simulink model "iot_casestudy_1_32"  (R2023a)
settings: Solver=VariableStepAuto  StartTime=0.0  StopTime=3.0  RelTol=1e-3
undefined symbols (not defined in the file or in its folder): m, n
(part 2 of 3)

== stateflow chart iot_casestudy_1_32/CameraScheduler4 ==
  settings: updateMethod=CONTINUOUS  executeAtInitialization=1
  state Main
    entry:
    dt=timer_array[i];
  (default) -> Main : {i=1;dt=0;}
  Main -> Main : after(dt,msec){i=i+1;send(schedule_driver);send(schedule_control);}
  data: timer_array input; schedule_driver output double; schedule_control output double; dt local double; dt2 local double; i output double =0.0

== stateflow chart iot_casestudy_1_32/CameraScheduler5 ==
  settings: updateMethod=CONTINUOUS  executeAtInitialization=1
  state Main
    entry:
    dt=timer_array[i];
  (default) -> Main : {i=0;dt=0;}
  Main -> Main : after(dt,msec){i=i+1;send(schedule_driver);send(schedule_control);}
  data: timer_array input; i local double; schedule_driver output double; schedule_control output double; dt local double

== stateflow chart iot_casestudy_1_32/CameraScheduler6 ==
  settings: updateMethod=CONTINUOUS  executeAtInitialization=1
  state Main
    entry:
    dt=timer_array[i];
  (default) -> Main : {i=1;dt=0;}
  Main -> Main : after(dt,msec){i=i+1;send(schedule_driver);send(schedule_control);}
  data: timer_array input; schedule_driver output double; schedule_control output double; dt local double; dt2 local double; i output double =0.0

== stateflow chart iot_casestudy_1_32/CameraScheduler7 ==
  settings: updateMethod=CONTINUOUS  executeAtInitialization=1
  state Main
    entry:
    dt=timer_array[i];
  (default) -> Main : {i=0;dt=0;}
  Main -> Main : after(dt,msec){i=i+1;send(schedule_driver);send(schedule_control);}
  data: timer_array input; i local double; schedule_driver output double; schedule_control output double; dt local double

== stateflow chart iot_casestudy_1_32/CameraControl10 ==
  settings: updateMethod=CONTINUOUS
  state Operation
    state RequestHangling [parallel]
      settings: executionOrder=1
      state Operation1
      (default) -> Operation1 : {image_request=1;}
      Operation1 -> Operation1 : schedule{image_request=1;}
    state ImageMessaging [parallel]
      settings: executionOrder=2
      state Operation2
        entry:
        validity=isvalid(imageIn);
      (default) -> Operation2 : {i=1;}
      (junction 28) -> Operation2 [order 1] : [validity==1]
          | {receive(imageIn);i = i + 1;
          | imageOut.data=imageIn.data
          | send(imageOut);}
      (junction 28) -> Operation2 [order 2] : {i = i + 1;receive(imageIn);}
      (junction 19) -> (junction 28) [order 1] : [network_faults(i)==0]
      (junction 19) -> Operation2 [order 2] : {receive(imageIn);i = i + 1;}
      Operation2 -> (junction 19) : schedule
  (default) -> Operation
  data: image_request output; imageIn input; i local; network_faults input; imageOut output; schedule input; validity local

== stateflow chart iot_casestudy_1_32/CameraControl11 ==
  settings: updateMethod=CONTINUOUS
  state Operation
    state RequestHangling [parallel]
      settings: executionOrder=1
      note: {image_request=1;}
      state Operation1
      (default) -> Operation1
      Operation1 -> Operation1 : schedule{image_request=1;}
    state ImageMessaging [parallel]
      settings: executionOrder=2
      state Operation2
        entry:
        validity=isvalid(imageIn);
      (default) -> Operation2 : {i=1;}
      (junction 29) -> Operation2 [order 1] : [isvalid(imageIn)==1]
          | {receive(imageIn);i = i + 1;
          | imageOut.data=imageIn.data;
          | send(imageOut);}
      (junction 19) -> Operation2 [order 2] : {receive(imageIn);i = i + 1;}
      Operation2 -> (junction 19) : schedule
      (junction 29) -> Operation2 [order 2] : {i = i + 1;receive(imageIn);}
      (junction 19) -> (junction 29) [order 1] : [network_faults(i)==0]
  (default) -> Operation
  data: image_request output; imageIn input; i local; network_faults input; imageOut output; schedule input; validity local

== stateflow chart iot_casestudy_1_32/CameraControl12 ==
  settings: updateMethod=CONTINUOUS
  state Operation
    state RequestHangling [parallel]
      settings: executionOrder=1
      state Operation1
      (default) -> Operation1 : {image_request=1;}
      Operation1 -> Operation1 : schedule{image_request=1;}
    state ImageMessaging [parallel]
      settings: executionOrder=2
      state Operation2
        entry:
        validity=isvalid(imageIn);
      (default) -> Operation2 : {i=1;}
      (junction 28) -> Operation2 [order 1] : [validity==1]
          | {receive(imageIn);i = i + 1;
          | imageOut.data=imageIn.data
          | send(imageOut);}
      (junction 28) -> Operation2 [order 2] : {i = i + 1;receive(imageIn);}
      (junction 19) -> (junction 28) [order 1] : [network_faults(i)==0]
      (junction 19) -> Operation2 [order 2] : {receive(imageIn);i = i + 1;}
      Operation2 -> (junction 19) : schedule
  (default) -> Operation
  data: image_request output; imageIn input; i local; network_faults input; imageOut output; schedule input; validity local

== stateflow chart iot_casestudy_1_32/CameraControl13 ==
  settings: updateMethod=CONTINUOUS
  state Operation
    state RequestHangling [parallel]
      settings: executionOrder=1
      note: {image_request=1;}
      state Operation1
      (default) -> Operation1
      Operation1 -> Operation1 : schedule{image_request=1;}
    state ImageMessaging [parallel]
      settings: executionOrder=2
      state Operation2
        entry:
        validity=isvalid(imageIn);
      (default) -> Operation2 : {i=1;}
      (junction 29) -> Operation2 [order 1] : [isvalid(imageIn)==1]
          | {receive(imageIn);i = i + 1;
          | imageOut.data=imageIn.data;
          | send(imageOut);}
      (junction 19) -> Operation2 [order 2] : {receive(imageIn);i = i + 1;}
      Operation2 -> (junction 19) : schedule
      (junction 29) -> Operation2 [order 2] : {i = i + 1;receive(imageIn);}
      (junction 19) -> (junction 29) [order 1] : [network_faults(i)==0]
  (default) -> Operation
  data: image_request output; imageIn input; i local; network_faults input; imageOut output; schedule input; validity local

== stateflow chart iot_casestudy_1_32/CameraControl14 ==
  settings: updateMethod=CONTINUOUS
  state Operation
    state RequestHangling [parallel]
      settings: executionOrder=1
      state Operation1
      (default) -> Operation1 : {image_request=1;}
      Operation1 -> Operation1 : schedule{image_request=1;}
    state ImageMessaging [parallel]
      settings: executionOrder=2
      state Operation2
        entry:
        validity=isvalid(imageIn);
      (default) -> Operation2 : {i=1;}
      (junction 28) -> Operation2 [order 1] : [validity==1]
          | {receive(imageIn);i = i + 1;
          | imageOut.data=imageIn.data
          | send(imageOut);}
      (junction 28) -> Operation2 [order 2] : {i = i + 1;receive(imageIn);}
      (junction 19) -> (junction 28) [order 1] : [network_faults(i)==0]
      (junction 19) -> Operation2 [order 2] : {receive(imageIn);i = i + 1;}
      Operation2 -> (junction 19) : schedule
  (default) -> Operation
  data: image_request output; imageIn input; i local; network_faults input; imageOut output; schedule input; validity local

== stateflow chart iot_casestudy_1_32/CameraControl15 ==
  settings: updateMethod=CONTINUOUS
  state Operation
    state RequestHangling [parallel]
      settings: executionOrder=1
      note: {image_request=1;}
      state Operation1
      (default) -> Operation1
      Operation1 -> Operation1 : schedule{image_request=1;}
    state ImageMessaging [parallel]
      settings: executionOrder=2
      state Operation2
        entry:
        validity=isvalid(imageIn);
      (default) -> Operation2 : {i=1;}
      (junction 29) -> Operation2 [order 1] : [isvalid(imageIn)==1]
          | {receive(imageIn);i = i + 1;
          | imageOut.data=imageIn.data;
          | send(imageOut);}
      (junction 19) -> Operation2 [order 2] : {receive(imageIn);i = i + 1;}
      Operation2 -> (junction 19) : schedule
      (junction 29) -> Operation2 [order 2] : {i = i + 1;receive(imageIn);}
      (junction 19) -> (junction 29) [order 1] : [network_faults(i)==0]
  (default) -> Operation
  data: image_request output; imageIn input; i local; network_faults input; imageOut output; schedule input; validity local

== stateflow chart iot_casestudy_1_32/CameraControl8 ==
  settings: updateMethod=CONTINUOUS
  state Operation
    state RequestHangling [parallel]
      settings: executionOrder=1
      state Operation1
      (default) -> Operation1 : {image_request=1;}
      Operation1 -> Operation1 : schedule{image_request=1;}
    state ImageMessaging [parallel]
      settings: executionOrder=2
      state Operation2
        entry:
        validity=isvalid(imageIn);
      (default) -> Operation2 : {i=1;}
      (junction 28) -> Operation2 [order 1] : [validity==1]
          | {receive(imageIn);i = i + 1;
          | imageOut.data=imageIn.data
          | send(imageOut);}
      (junction 28) -> Operation2 [order 2] : {i = i + 1;receive(imageIn);}
      (junction 19) -> (junction 28) [order 1] : [network_faults(i)==0]
      (junction 19) -> Operation2 [order 2] : {receive(imageIn);i = i + 1;}
      Operation2 -> (junction 19) : schedule
  (default) -> Operation
  data: image_request output; imageIn input; i local; network_faults input; imageOut output; schedule input; validity local

== stateflow chart iot_casestudy_1_32/CameraControl9 ==
  settings: updateMethod=CONTINUOUS
  state Operation
    state RequestHangling [parallel]
      settings: executionOrder=1
      note: {image_request=1;}
      state Operation1
      (default) -> Operation1
      Operation1 -> Operation1 : schedule{image_request=1;}
    state ImageMessaging [parallel]
      settings: executionOrder=2
      state Operation2
        entry:
        validity=isvalid(imageIn);
      (default) -> Operation2 : {i=1;}
      (junction 29) -> Operation2 [order 1] : [isvalid(imageIn)==1]
          | {receive(imageIn);i = i + 1;
          | imageOut.data=imageIn.data;
          | send(imageOut);}
      (junction 19) -> Operation2 [order 2] : {receive(imageIn);i = i + 1;}
      Operation2 -> (junction 19) : schedule
      (junction 29) -> Operation2 [order 2] : {i = i + 1;receive(imageIn);}
      (junction 19) -> (junction 29) [order 1] : [network_faults(i)==0]
  (default) -> Operation
  data: image_request output; imageIn input; i local; network_faults input; imageOut output; schedule input; validity local

== stateflow chart iot_casestudy_1_32/CameraDriver10 ==
  settings: updateMethod=CONTINUOUS
  state Operation
    state CarVisibility [parallel]
      settings: executionOrder=1
      state NoCar
        entry: car=0;
      state Car
        entry: car=1;
      (default) -> NoCar
      NoCar -> Car : [traffic_state==1]
      Car -> NoCar : [traffic_state==0]
    state DriverOperation [parallel]
      settings: executionOrder=2
      state Main
      (default) -> Main : {i=1;}
      Main -> (junction 22) : schedule[image_request]
      (junction 22) -> Main [order 2] : {image.data=0;
          | send(image);i = i + 1;}
      (junction 22) -> Main [order 1] : [(car==1)&&(blurryness(i)==1)]
          | {image.data=1;i = i + 1;send(image);}
  data: image_request input; traffic_state input; blurryness input; image output; car local; i local; schedule input

== stateflow chart iot_casestudy_1_32/CameraDriver11 ==
  settings: updateMethod=CONTINUOUS
  state Operation
    state CarVisibility [parallel]
      settings: executionOrder=1
      state NoCar
        entry: car=0;
      state Car
        entry: car=1;
      (default) -> NoCar
      NoCar -> Car : [traffic_state==1]
      Car -> NoCar : [traffic_state==0]
    state DriverOperation [parallel]
      settings: executionOrder=2
      state Main
      (default) -> Main : {i=1;}
      Main -> (junction 22) : schedule
          | [image_request]
      (junction 22) -> Main [order 1] : [(car==1)&&(blurryness(i)==1)]
          | {image.data=1;send(image);i = i + 1;}
      (junction 22) -> Main [order 2] : {image.data=0;
          | send(image);i = i + 1;}
  data: image_request input; traffic_state input; blurryness input; image output; car local; i local; schedule input

== stateflow chart iot_casestudy_1_32/CameraDriver12 ==
  settings: updateMethod=CONTINUOUS
  state Operation
    state CarVisibility [parallel]
      settings: executionOrder=1
      state NoCar
        entry: car=0;
      state Car
        entry: car=1;
      (default) -> NoCar
      NoCar -> Car : [traffic_state==1]
      Car -> NoCar : [traffic_state==0]
    state DriverOperation [parallel]
      settings: executionOrder=2
      state Main
      (default) -> Main : {i=1;}
      Main -> (junction 22) : schedule[image_request]
      (junction 22) -> Main [order 2] : {image.data=0;
          | send(image);i = i + 1;}
      (junction 22) -> Main [order 1] : [(car==1)&&(blurryness(i)==1)]
          | {image.data=1;i = i + 1;send(image);}
  data: image_request input; traffic_state input; blurryness input; image output; car local; i local; schedule input

== stateflow chart iot_casestudy_1_32/CameraDriver13 ==
  settings: updateMethod=CONTINUOUS
  state Operation
    state CarVisibility [parallel]
      settings: executionOrder=1
      state NoCar
        entry: car=0;
      state Car
        entry: car=1;
      (default) -> NoCar
      NoCar -> Car : [traffic_state==1]
      Car -> NoCar : [traffic_state==0]
    state DriverOperation [parallel]
      settings: executionOrder=2
      state Main
      (default) -> Main : {i=1;}
      Main -> (junction 22) : schedule
          | [image_request]
      (junction 22) -> Main [order 1] : [(car==1)&&(blurryness(i)==1)]
          | {image.data=1;send(image);i = i + 1;}
      (junction 22) -> Main [order 2] : {image.data=0;
          | send(image);i = i + 1;}
  data: image_request input; traffic_state input; blurryness input; image output; car local; i local; schedule input

== stateflow chart iot_casestudy_1_32/CameraDriver14 ==
  settings: updateMethod=CONTINUOUS
  state Operation
    state CarVisibility [parallel]
      settings: executionOrder=1
      state NoCar
        entry: car=0;
      state Car
        entry: car=1;
      (default) -> NoCar
      NoCar -> Car : [traffic_state==1]
      Car -> NoCar : [traffic_state==0]
    state DriverOperation [parallel]
      settings: executionOrder=2
      state Main
      (default) -> Main : {i=1;}
      Main -> (junction 22) : schedule[image_request]
      (junction 22) -> Main [order 2] : {image.data=0;
          | send(image);i = i + 1;}
      (junction 22) -> Main [order 1] : [(car==1)&&(blurryness(i)==1)]
          | {image.data=1;i = i + 1;send(image);}
  data: image_request input; traffic_state input; blurryness input; image output; car local; i local; schedule input

== stateflow chart iot_casestudy_1_32/CameraDriver15 ==
  settings: updateMethod=CONTINUOUS
  state Operation
    state CarVisibility [parallel]
      settings: executionOrder=1
      state NoCar
        entry: car=0;
      state Car
        entry: car=1;
      (default) -> NoCar
      NoCar -> Car : [traffic_state==1]
      Car -> NoCar : [traffic_state==0]
    state DriverOperation [parallel]
      settings: executionOrder=2
      state Main
      (default) -> Main : {i=1;}
      Main -> (junction 22) : schedule
          | [image_request]
      (junction 22) -> Main [order 1] : [(car==1)&&(blurryness(i)==1)]
          | {image.data=1;send(image);i = i + 1;}
      (junction 22) -> Main [order 2] : {image.data=0;
          | send(image);i = i + 1;}
  data: image_request input; traffic_state input; blurryness input; image output; car local; i local; schedule input

== stateflow chart iot_casestudy_1_32/CameraDriver8 ==
  settings: updateMethod=CONTINUOUS
  state Operation
    state CarVisibility [parallel]
      settings: executionOrder=1
      state NoCar
        entry: car=0;
      state Car
        entry: car=1;
      (default) -> NoCar
      NoCar -> Car : [traffic_state==1]
      Car -> NoCar : [traffic_state==0]
    state DriverOperation [parallel]
      settings: executionOrder=2
      state Main
      (default) -> Main : {i=1;}
      Main -> (junction 22) : schedule[image_request]
      (junction 22) -> Main [order 2] : {image.data=0;
          | send(image);i = i + 1;}
      (junction 22) -> Main [order 1] : [(car==1)&&(blurryness(i)==1)]
          | {image.data=1;i = i + 1;send(image);}
  data: image_request input; traffic_state input; blurryness input; image output; car local; i local; schedule input

== stateflow chart iot_casestudy_1_32/CameraDriver9 ==
  settings: updateMethod=CONTINUOUS
  state Operation
    state CarVisibility [parallel]
      settings: executionOrder=1
      state NoCar
        entry: car=0;
      state Car
        entry: car=1;
      (default) -> NoCar
      NoCar -> Car : [traffic_state==1]
      Car -> NoCar : [traffic_state==0]
    state DriverOperation [parallel]
      settings: executionOrder=2
      state Main
      (default) -> Main : {i=1;}
      Main -> (junction 22) : schedule
          | [image_request]
      (junction 22) -> Main [order 1] : [(car==1)&&(blurryness(i)==1)]
          | {image.data=1;send(image);i = i + 1;}
      (junction 22) -> Main [order 2] : {image.data=0;
          | send(image);i = i + 1;}
  data: image_request input; traffic_state input; blurryness input; image output; car local; i local; schedule input

== stateflow chart iot_casestudy_1_32/CameraScheduler10 ==
  settings: updateMethod=CONTINUOUS  executeAtInitialization=1
  state Main
    entry:
    dt=timer_array[i];
  (default) -> Main : {i=1;dt=0;}
  Main -> Main : after(dt,msec){i=i+1;send(schedule_driver);send(schedule_control);}
  data: timer_array input; schedule_driver output double; schedule_control output double; dt local double; dt2 local double; i local double =0.0

== stateflow chart iot_casestudy_1_32/CameraScheduler11 ==
  settings: updateMethod=CONTINUOUS  executeAtInitialization=1
  state Main
    entry:
    dt=timer_array[i];
  (default) -> Main : {i=0;dt=0;}
  Main -> Main : after(dt,msec){i=i+1;send(schedule_driver);send(schedule_control);}
  data: timer_array input; i local double; schedule_driver output double; schedule_control output double; dt local double

== stateflow chart iot_casestudy_1_32/CameraScheduler12 ==
  settings: updateMethod=CONTINUOUS  executeAtInitialization=1
  state Main
    entry:
    dt=timer_array[i];
  (default) -> Main : {i=1;dt=0;}
  Main -> Main : after(dt,msec){i=i+1;send(schedule_driver);send(schedule_control);}
  data: timer_array input; schedule_driver output double; schedule_control output double; dt local double; dt2 local double; i local double =0.0

== stateflow chart iot_casestudy_1_32/CameraScheduler13 ==
  settings: updateMethod=CONTINUOUS  executeAtInitialization=1
  state Main
    entry:
    dt=timer_array[i];
  (default) -> Main : {i=0;dt=0;}
  Main -> Main : after(dt,msec){i=i+1;send(schedule_driver);send(schedule_control);}
  data: timer_array input; i local double; schedule_driver output double; schedule_control output double; dt local double

== stateflow chart iot_casestudy_1_32/CameraScheduler14 ==
  settings: updateMethod=CONTINUOUS  executeAtInitialization=1
  state Main
    entry:
    dt=timer_array[i];
  (default) -> Main : {i=1;dt=0;}
  Main -> Main : after(dt,msec){i=i+1;send(schedule_driver);send(schedule_control);}
  data: timer_array input; schedule_driver output double; schedule_control output double; dt local double; dt2 local double; i local double =0.0

== stateflow chart iot_casestudy_1_32/CameraScheduler15 ==
  settings: updateMethod=CONTINUOUS  executeAtInitialization=1
  state Main
    entry:
    dt=timer_array[i];
  (default) -> Main : {i=0;dt=0;}
  Main -> Main : after(dt,msec){i=i+1;send(schedule_driver);send(schedule_control);}
  data: timer_array input; i local double; schedule_driver output double; schedule_control output double; dt local double

== stateflow chart iot_casestudy_1_32/CameraScheduler8 ==
  settings: updateMethod=CONTINUOUS  executeAtInitialization=1
  state Main
    entry:
    dt=timer_array[i];
  (default) -> Main : {i=1;dt=0;}
  Main -> Main : after(dt,msec){i=i+1;send(schedule_driver);send(schedule_control);}
  data: timer_array input; schedule_driver output double; schedule_control output double; dt local double; dt2 local double; i local double =0.0

== stateflow chart iot_casestudy_1_32/CameraScheduler9 ==
  settings: updateMethod=CONTINUOUS  executeAtInitialization=1
  state Main
    entry:
    dt=timer_array[i];
  (default) -> Main : {i=0;dt=0;}
  Main -> Main : after(dt,msec){i=i+1;send(schedule_driver);send(schedule_control);}
  data: timer_array input; i local double; schedule_driver output double; schedule_control output double; dt local double

== stateflow chart iot_casestudy_1_32/CameraControl16 ==
  settings: updateMethod=CONTINUOUS
  state Operation
    state RequestHangling [parallel]
      settings: executionOrder=1
      state Operation1
      (default) -> Operation1 : {image_request=1;}
      Operation1 -> Operation1 : schedule{image_request=1;}
    state ImageMessaging [parallel]
      settings: executionOrder=2
      state Operation2
        entry:
        validity=isvalid(imageIn);
      (default) -> Operation2 : {i=1;}
      (junction 28) -> Operation2 [order 1] : [validity==1]
          | {receive(imageIn);i = i + 1;
          | imageOut.data=imageIn.data
          | send(imageOut);}
      (junction 28) -> Operation2 [order 2] : {i = i + 1;receive(imageIn);}
      (junction 19) -> (junction 28) [order 1] : [network_faults(i)==0]
      (junction 19) -> Operation2 [order 2] : {receive(imageIn);i = i + 1;}
      Operation2 -> (junction 19) : schedule
  (default) -> Operation
  data: image_request output; imageIn input; i local; network_faults input; imageOut output; schedule input; validity local

== stateflow chart iot_casestudy_1_32/CameraControl17 ==
  settings: updateMethod=CONTINUOUS
  state Operation
    state RequestHangling [parallel]
      settings: executionOrder=1
      note: {image_request=1;}
      state Operation1
      (default) -> Operation1
      Operation1 -> Operation1 : schedule{image_request=1;}
    state ImageMessaging [parallel]
      settings: executionOrder=2
      state Operation2
        entry:
        validity=isvalid(imageIn);
      (default) -> Operation2 : {i=1;}
      (junction 29) -> Operation2 [order 1] : [isvalid(imageIn)==1]
          | {receive(imageIn);i = i + 1;
          | imageOut.data=imageIn.data;
          | send(imageOut);}
      (junction 19) -> Operation2 [order 2] : {receive(imageIn);i = i + 1;}
      Operation2 -> (junction 19) : schedule
      (junction 29) -> Operation2 [order 2] : {i = i + 1;receive(imageIn);}
      (junction 19) -> (junction 29) [order 1] : [network_faults(i)==0]
  (default) -> Operation
  data: image_request output; imageIn input; i local; network_faults input; imageOut output; schedule input; validity local

== stateflow chart iot_casestudy_1_32/CameraControl18 ==
  settings: updateMethod=CONTINUOUS
  state Operation
    state RequestHangling [parallel]
      settings: executionOrder=1
      state Operation1
      (default) -> Operation1 : {image_request=1;}
      Operation1 -> Operation1 : schedule{image_request=1;}
    state ImageMessaging [parallel]
      settings: executionOrder=2
      state Operation2
        entry:
        validity=isvalid(imageIn);
      (default) -> Operation2 : {i=1;}
      (junction 28) -> Operation2 [order 1] : [validity==1]
          | {receive(imageIn);i = i + 1;
          | imageOut.data=imageIn.data
          | send(imageOut);}
      (junction 28) -> Operation2 [order 2] : {i = i + 1;receive(imageIn);}
      (junction 19) -> (junction 28) [order 1] : [network_faults(i)==0]
      (junction 19) -> Operation2 [order 2] : {receive(imageIn);i = i + 1;}
      Operation2 -> (junction 19) : schedule
  (default) -> Operation
  data: image_request output; imageIn input; i local; network_faults input; imageOut output; schedule input; validity local

== stateflow chart iot_casestudy_1_32/CameraControl19 ==
  settings: updateMethod=CONTINUOUS
  state Operation
    state RequestHangling [parallel]
      settings: executionOrder=1
      note: {image_request=1;}
      state Operation1
      (default) -> Operation1
      Operation1 -> Operation1 : schedule{image_request=1;}
    state ImageMessaging [parallel]
      settings: executionOrder=2
      state Operation2
        entry:
        validity=isvalid(imageIn);
      (default) -> Operation2 : {i=1;}
      (junction 29) -> Operation2 [order 1] : [isvalid(imageIn)==1]
          | {receive(imageIn);i = i + 1;
          | imageOut.data=imageIn.data;
          | send(imageOut);}
      (junction 19) -> Operation2 [order 2] : {receive(imageIn);i = i + 1;}
      Operation2 -> (junction 19) : schedule
      (junction 29) -> Operation2 [order 2] : {i = i + 1;receive(imageIn);}
      (junction 19) -> (junction 29) [order 1] : [network_faults(i)==0]
  (default) -> Operation
  data: image_request output; imageIn input; i local; network_faults input; imageOut output; schedule input; validity local

== stateflow chart iot_casestudy_1_32/CameraControl20 ==
  settings: updateMethod=CONTINUOUS
  state Operation
    state RequestHangling [parallel]
      settings: executionOrder=1
      state Operation1
      (default) -> Operation1 : {image_request=1;}
      Operation1 -> Operation1 : schedule{image_request=1;}
    state ImageMessaging [parallel]
      settings: executionOrder=2
      state Operation2
        entry:
        validity=isvalid(imageIn);
      (default) -> Operation2 : {i=1;}
      (junction 28) -> Operation2 [order 1] : [validity==1]
          | {receive(imageIn);i = i + 1;
          | imageOut.data=imageIn.data
          | send(imageOut);}
      (junction 28) -> Operation2 [order 2] : {i = i + 1;receive(imageIn);}
      (junction 19) -> (junction 28) [order 1] : [network_faults(i)==0]
      (junction 19) -> Operation2 [order 2] : {receive(imageIn);i = i + 1;}
      Operation2 -> (junction 19) : schedule
  (default) -> Operation
  data: image_request output; imageIn input; i local; network_faults input; imageOut output; schedule input; validity local

== stateflow chart iot_casestudy_1_32/CameraControl21 ==
  settings: updateMethod=CONTINUOUS
  state Operation
    state RequestHangling [parallel]
      settings: executionOrder=1
      note: {image_request=1;}
      state Operation1
      (default) -> Operation1
      Operation1 -> Operation1 : schedule{image_request=1;}
    state ImageMessaging [parallel]
      settings: executionOrder=2
      state Operation2
        entry:
        validity=isvalid(imageIn);
      (default) -> Operation2 : {i=1;}
      (junction 29) -> Operation2 [order 1] : [isvalid(imageIn)==1]
          | {receive(imageIn);i = i + 1;
          | imageOut.data=imageIn.data;
          | send(imageOut);}
      (junction 19) -> Operation2 [order 2] : {receive(imageIn);i = i + 1;}
      Operation2 -> (junction 19) : schedule
      (junction 29) -> Operation2 [order 2] : {i = i + 1;receive(imageIn);}
      (junction 19) -> (junction 29) [order 1] : [network_faults(i)==0]
  (default) -> Operation
  data: image_request output; imageIn input; i local; network_faults input; imageOut output; schedule input; validity local

== stateflow chart iot_casestudy_1_32/CameraControl22 ==
  settings: updateMethod=CONTINUOUS
  state Operation
    state RequestHangling [parallel]
      settings: executionOrder=1
      state Operation1
      (default) -> Operation1 : {image_request=1;}
      Operation1 -> Operation1 : schedule{image_request=1;}
    state ImageMessaging [parallel]
      settings: executionOrder=2
      state Operation2
        entry:
        validity=isvalid(imageIn);
      (default) -> Operation2 : {i=1;}
      (junction 28) -> Operation2 [order 1] : [validity==1]
          | {receive(imageIn);i = i + 1;
          | imageOut.data=imageIn.data
          | send(imageOut);}
      (junction 28) -> Operation2 [order 2] : {i = i + 1;receive(imageIn);}
      (junction 19) -> (junction 28) [order 1] : [network_faults(i)==0]
      (junction 19) -> Operation2 [order 2] : {receive(imageIn);i = i + 1;}
      Operation2 -> (junction 19) : schedule
  (default) -> Operation
  data: image_request output; imageIn input; i local; network_faults input; imageOut output; schedule input; validity local

== stateflow chart iot_casestudy_1_32/CameraControl23 ==
  settings: updateMethod=CONTINUOUS
  state Operation
    state RequestHangling [parallel]
      settings: executionOrder=1
      note: {image_request=1;}
      state Operation1
      (default) -> Operation1
      Operation1 -> Operation1 : schedule{image_request=1;}
    state ImageMessaging [parallel]
      settings: executionOrder=2
      state Operation2
        entry:
        validity=isvalid(imageIn);
      (default) -> Operation2 : {i=1;}
      (junction 29) -> Operation2 [order 1] : [isvalid(imageIn)==1]
          | {receive(imageIn);i = i + 1;
          | imageOut.data=imageIn.data;
          | send(imageOut);}
      (junction 19) -> Operation2 [order 2] : {receive(imageIn);i = i + 1;}
      Operation2 -> (junction 19) : schedule
      (junction 29) -> Operation2 [order 2] : {i = i + 1;receive(imageIn);}
      (junction 19) -> (junction 29) [order 1] : [network_faults(i)==0]
  (default) -> Operation
  data: image_request output; imageIn input; i local; network_faults input; imageOut output; schedule input; validity local

== stateflow chart iot_casestudy_1_32/CameraControl24 ==
  settings: updateMethod=CONTINUOUS
  state Operation
    state RequestHangling [parallel]
      settings: executionOrder=1
      state Operation1
      (default) -> Operation1 : {image_request=1;}
      Operation1 -> Operation1 : schedule{image_request=1;}
    state ImageMessaging [parallel]
      settings: executionOrder=2
      state Operation2
        entry:
        validity=isvalid(imageIn);
      (default) -> Operation2 : {i=1;}
      (junction 28) -> Operation2 [order 1] : [validity==1]
          | {receive(imageIn);i = i + 1;
          | imageOut.data=imageIn.data
          | send(imageOut);}
      (junction 28) -> Operation2 [order 2] : {i = i + 1;receive(imageIn);}
      (junction 19) -> (junction 28) [order 1] : [network_faults(i)==0]
      (junction 19) -> Operation2 [order 2] : {receive(imageIn);i = i + 1;}
      Operation2 -> (junction 19) : schedule
  (default) -> Operation
  data: image_request output; imageIn input; i local; network_faults input; imageOut output; schedule input; validity local

== stateflow chart iot_casestudy_1_32/CameraControl25 ==
  settings: updateMethod=CONTINUOUS
  state Operation
    state RequestHangling [parallel]
      settings: executionOrder=1
      note: {image_request=1;}
      state Operation1
      (default) -> Operation1
      Operation1 -> Operation1 : schedule{image_request=1;}
    state ImageMessaging [parallel]
      settings: executionOrder=2
      state Operation2
        entry:
        validity=isvalid(imageIn);
      (default) -> Operation2 : {i=1;}
      (junction 29) -> Operation2 [order 1] : [isvalid(imageIn)==1]
          | {receive(imageIn);i = i + 1;
          | imageOut.data=imageIn.data;
          | send(imageOut);}
      (junction 19) -> Operation2 [order 2] : {receive(imageIn);i = i + 1;}
      Operation2 -> (junction 19) : schedule
      (junction 29) -> Operation2 [order 2] : {i = i + 1;receive(imageIn);}
      (junction 19) -> (junction 29) [order 1] : [network_faults(i)==0]
  (default) -> Operation
  data: image_request output; imageIn input; i local; network_faults input; imageOut output; schedule input; validity local

== stateflow chart iot_casestudy_1_32/CameraControl26 ==
  settings: updateMethod=CONTINUOUS
  state Operation
    state RequestHangling [parallel]
      settings: executionOrder=1
      state Operation1
      (default) -> Operation1 : {image_request=1;}
      Operation1 -> Operation1 : schedule{image_request=1;}
    state ImageMessaging [parallel]
      settings: executionOrder=2
      state Operation2
        entry:
        validity=isvalid(imageIn);
      (default) -> Operation2 : {i=1;}
      (junction 28) -> Operation2 [order 1] : [validity==1]
          | {receive(imageIn);i = i + 1;
          | imageOut.data=imageIn.data
          | send(imageOut);}
      (junction 28) -> Operation2 [order 2] : {i = i + 1;receive(imageIn);}
      (junction 19) -> (junction 28) [order 1] : [network_faults(i)==0]
      (junction 19) -> Operation2 [order 2] : {receive(imageIn);i = i + 1;}
      Operation2 -> (junction 19) : schedule
  (default) -> Operation
  data: image_request output; imageIn input; i local; network_faults input; imageOut output; schedule input; validity local

== stateflow chart iot_casestudy_1_32/CameraControl27 ==
  settings: updateMethod=CONTINUOUS
  state Operation
    state RequestHangling [parallel]
      settings: executionOrder=1
      note: {image_request=1;}
      state Operation1
      (default) -> Operation1
      Operation1 -> Operation1 : schedule{image_request=1;}
    state ImageMessaging [parallel]
      settings: executionOrder=2
      state Operation2
        entry:
        validity=isvalid(imageIn);
      (default) -> Operation2 : {i=1;}
      (junction 29) -> Operation2 [order 1] : [isvalid(imageIn)==1]
          | {receive(imageIn);i = i + 1;
          | imageOut.data=imageIn.data;
          | send(imageOut);}
      (junction 19) -> Operation2 [order 2] : {receive(imageIn);i = i + 1;}
      Operation2 -> (junction 19) : schedule
      (junction 29) -> Operation2 [order 2] : {i = i + 1;receive(imageIn);}
      (junction 19) -> (junction 29) [order 1] : [network_faults(i)==0]
  (default) -> Operation
  data: image_request output; imageIn input; i local; network_faults input; imageOut output; schedule input; validity local

== stateflow chart iot_casestudy_1_32/CameraControl28 ==
  settings: updateMethod=CONTINUOUS
  state Operation
    state RequestHangling [parallel]
      settings: executionOrder=1
      state Operation1
      (default) -> Operation1 : {image_request=1;}
      Operation1 -> Operation1 : schedule{image_request=1;}
    state ImageMessaging [parallel]
      settings: executionOrder=2
      state Operation2
        entry:
        validity=isvalid(imageIn);
      (default) -> Operation2 : {i=1;}
      (junction 28) -> Operation2 [order 1] : [validity==1]
          | {receive(imageIn);i = i + 1;
          | imageOut.data=imageIn.data
          | send(imageOut);}
      (junction 28) -> Operation2 [order 2] : {i = i + 1;receive(imageIn);}
      (junction 19) -> (junction 28) [order 1] : [network_faults(i)==0]
      (junction 19) -> Operation2 [order 2] : {receive(imageIn);i = i + 1;}
      Operation2 -> (junction 19) : schedule
  (default) -> Operation
  data: image_request output; imageIn input; i local; network_faults input; imageOut output; schedule input; validity local

== stateflow chart iot_casestudy_1_32/CameraControl29 ==
  settings: updateMethod=CONTINUOUS
  state Operation
    state RequestHangling [parallel]
      settings: executionOrder=1
      note: {image_request=1;}
      state Operation1
      (default) -> Operation1
      Operation1 -> Operation1 : schedule{image_request=1;}
    state ImageMessaging [parallel]
      settings: executionOrder=2
      state Operation2
        entry:
        validity=isvalid(imageIn);
      (default) -> Operation2 : {i=1;}
      (junction 29) -> Operation2 [order 1] : [isvalid(imageIn)==1]
          | {receive(imageIn);i = i + 1;
          | imageOut.data=imageIn.data;
          | send(imageOut);}
      (junction 19) -> Operation2 [order 2] : {receive(imageIn);i = i + 1;}
      Operation2 -> (junction 19) : schedule
      (junction 29) -> Operation2 [order 2] : {i = i + 1;receive(imageIn);}
      (junction 19) -> (junction 29) [order 1] : [network_faults(i)==0]
  (default) -> Operation
  data: image_request output; imageIn input; i local; network_faults input; imageOut output; schedule input; validity local

== stateflow chart iot_casestudy_1_32/CameraControl30 ==
  settings: updateMethod=CONTINUOUS
  state Operation
    state RequestHangling [parallel]
      settings: executionOrder=1
      state Operation1
      (default) -> Operation1 : {image_request=1;}
      Operation1 -> Operation1 : schedule{image_request=1;}
    state ImageMessaging [parallel]
      settings: executionOrder=2
      state Operation2
        entry:
        validity=isvalid(imageIn);
      (default) -> Operation2 : {i=1;}
      (junction 28) -> Operation2 [order 1] : [validity==1]
          | {receive(imageIn);i = i + 1;
          | imageOut.data=imageIn.data
          | send(imageOut);}
      (junction 28) -> Operation2 [order 2] : {i = i + 1;receive(imageIn);}
      (junction 19) -> (junction 28) [order 1] : [network_faults(i)==0]
      (junction 19) -> Operation2 [order 2] : {receive(imageIn);i = i + 1;}
      Operation2 -> (junction 19) : schedule
  (default) -> Operation
  data: image_request output; imageIn input; i local; network_faults input; imageOut output; schedule input; validity local

== stateflow chart iot_casestudy_1_32/CameraControl31 ==
  settings: updateMethod=CONTINUOUS
  state Operation
    state RequestHangling [parallel]
      settings: executionOrder=1
      note: {image_request=1;}
      state Operation1
      (default) -> Operation1
      Operation1 -> Operation1 : schedule{image_request=1;}
    state ImageMessaging [parallel]
      settings: executionOrder=2
      state Operation2
        entry:
        validity=isvalid(imageIn);
      (default) -> Operation2 : {i=1;}
      (junction 29) -> Operation2 [order 1] : [isvalid(imageIn)==1]
          | {receive(imageIn);i = i + 1;
          | imageOut.data=imageIn.data;
          | send(imageOut);}
      (junction 19) -> Operation2 [order 2] : {receive(imageIn);i = i + 1;}
      Operation2 -> (junction 19) : schedule
      (junction 29) -> Operation2 [order 2] : {i = i + 1;receive(imageIn);}
      (junction 19) -> (junction 29) [order 1] : [network_faults(i)==0]
  (default) -> Operation
  data: image_request output; imageIn input; i local; network_faults input; imageOut output; schedule input; validity local

== stateflow chart iot_casestudy_1_32/CameraDriver16 ==
  settings: updateMethod=CONTINUOUS
  state Operation
    state CarVisibility [parallel]
      settings: executionOrder=1
      state NoCar
        entry: car=0;
      state Car
        entry: car=1;
      (default) -> NoCar
      NoCar -> Car : [traffic_state==1]
      Car -> NoCar : [traffic_state==0]
    state DriverOperation [parallel]
      settings: executionOrder=2
      state Main
      (default) -> Main : {i=1;}
      Main -> (junction 22) : schedule[image_request]
      (junction 22) -> Main [order 2] : {image.data=0;
          | send(image);i = i + 1;}
      (junction 22) -> Main [order 1] : [(car==1)&&(blurryness(i)==1)]
          | {image.data=1;i = i + 1;send(image);}
  data: image_request input; traffic_state input; blurryness input; image output; car local; i local; schedule input

== stateflow chart iot_casestudy_1_32/CameraDriver17 ==
  settings: updateMethod=CONTINUOUS
  state Operation
    state CarVisibility [parallel]
      settings: executionOrder=1
      state NoCar
        entry: car=0;
      state Car
        entry: car=1;
      (default) -> NoCar
      NoCar -> Car : [traffic_state==1]
      Car -> NoCar : [traffic_state==0]
    state DriverOperation [parallel]
      settings: executionOrder=2
      state Main
      (default) -> Main : {i=1;}
      Main -> (junction 22) : schedule
          | [image_request]
      (junction 22) -> Main [order 1] : [(car==1)&&(blurryness(i)==1)]
          | {image.data=1;send(image);i = i + 1;}
      (junction 22) -> Main [order 2] : {image.data=0;
          | send(image);i = i + 1;}
  data: image_request input; traffic_state input; blurryness input; image output; car local; i local; schedule input

== stateflow chart iot_casestudy_1_32/CameraDriver18 ==
  settings: updateMethod=CONTINUOUS
  state Operation
    state CarVisibility [parallel]
      settings: executionOrder=1
      state NoCar
        entry: car=0;
      state Car
        entry: car=1;
      (default) -> NoCar
      NoCar -> Car : [traffic_state==1]
      Car -> NoCar : [traffic_state==0]
    state DriverOperation [parallel]
      settings: executionOrder=2
      state Main
      (default) -> Main : {i=1;}
      Main -> (junction 22) : schedule[image_request]
      (junction 22) -> Main [order 2] : {image.data=0;
          | send(image);i = i + 1;}
      (junction 22) -> Main [order 1] : [(car==1)&&(blurryness(i)==1)]
          | {image.data=1;i = i + 1;send(image);}
  data: image_request input; traffic_state input; blurryness input; image output; car local; i local; schedule input

== stateflow chart iot_casestudy_1_32/CameraDriver19 ==
  settings: updateMethod=CONTINUOUS
  state Operation
    state CarVisibility [parallel]
      settings: executionOrder=1
      state NoCar
        entry: car=0;
      state Car
        entry: car=1;
      (default) -> NoCar
      NoCar -> Car : [traffic_state==1]
      Car -> NoCar : [traffic_state==0]
    state DriverOperation [parallel]
      settings: executionOrder=2
      state Main
      (default) -> Main : {i=1;}
      Main -> (junction 22) : schedule
          | [image_request]
      (junction 22) -> Main [order 1] : [(car==1)&&(blurryness(i)==1)]
          | {image.data=1;send(image);i = i + 1;}
      (junction 22) -> Main [order 2] : {image.data=0;
          | send(image);i = i + 1;}
  data: image_request input; traffic_state input; blurryness input; image output; car local; i local; schedule input

== stateflow chart iot_casestudy_1_32/CameraDriver20 ==
  settings: updateMethod=CONTINUOUS
  state Operation
    state CarVisibility [parallel]
      settings: executionOrder=1
      state NoCar
        entry: car=0;
      state Car
        entry: car=1;
      (default) -> NoCar
      NoCar -> Car : [traffic_state==1]
      Car -> NoCar : [traffic_state==0]
    state DriverOperation [parallel]
      settings: executionOrder=2
      state Main
      (default) -> Main : {i=1;}
      Main -> (junction 22) : schedule[image_request]
      (junction 22) -> Main [order 2] : {image.data=0;
          | send(image);i = i + 1;}
      (junction 22) -> Main [order 1] : [(car==1)&&(blurryness(i)==1)]
          | {image.data=1;i = i + 1;send(image);}
  data: image_request input; traffic_state input; blurryness input; image output; car local; i local; schedule input

== stateflow chart iot_casestudy_1_32/CameraDriver21 ==
  settings: updateMethod=CONTINUOUS
  state Operation
    state CarVisibility [parallel]
      settings: executionOrder=1
      state NoCar
        entry: car=0;
      state Car
        entry: car=1;
      (default) -> NoCar
      NoCar -> Car : [traffic_state==1]
      Car -> NoCar : [traffic_state==0]
    state DriverOperation [parallel]
      settings: executionOrder=2
      state Main
      (default) -> Main : {i=1;}
      Main -> (junction 22) : schedule
          | [image_request]
      (junction 22) -> Main [order 1] : [(car==1)&&(blurryness(i)==1)]
          | {image.data=1;send(image);i = i + 1;}
      (junction 22) -> Main [order 2] : {image.data=0;
          | send(image);i = i + 1;}
  data: image_request input; traffic_state input; blurryness input; image output; car local; i local; schedule input

== stateflow chart iot_casestudy_1_32/CameraDriver22 ==
  settings: updateMethod=CONTINUOUS
  state Operation
    state CarVisibility [parallel]
      settings: executionOrder=1
      state NoCar
        entry: car=0;
      state Car
        entry: car=1;
      (default) -> NoCar
      NoCar -> Car : [traffic_state==1]
      Car -> NoCar : [traffic_state==0]
    state DriverOperation [parallel]
      settings: executionOrder=2
      state Main
      (default) -> Main : {i=1;}
      Main -> (junction 22) : schedule[image_request]
      (junction 22) -> Main [order 2] : {image.data=0;
          | send(image);i = i + 1;}
      (junction 22) -> Main [order 1] : [(car==1)&&(blurryness(i)==1)]
          | {image.data=1;i = i + 1;send(image);}
  data: image_request input; traffic_state input; blurryness input; image output; car local; i local; schedule input

== stateflow chart iot_casestudy_1_32/CameraDriver23 ==
  settings: updateMethod=CONTINUOUS
  state Operation
    state CarVisibility [parallel]
      settings: executionOrder=1
      state NoCar
        entry: car=0;
      state Car
        entry: car=1;
      (default) -> NoCar
      NoCar -> Car : [traffic_state==1]
      Car -> NoCar : [traffic_state==0]
    state DriverOperation [parallel]
      settings: executionOrder=2
      state Main
      (default) -> Main : {i=1;}
      Main -> (junction 22) : schedule
          | [image_request]
      (junction 22) -> Main [order 1] : [(car==1)&&(blurryness(i)==1)]
          | {image.data=1;send(image);i = i + 1;}
      (junction 22) -> Main [order 2] : {image.data=0;
          | send(image);i = i + 1;}
  data: image_request input; traffic_state input; blurryness input; image output; car local; i local; schedule input

== stateflow chart iot_casestudy_1_32/CameraDriver24 ==
  settings: updateMethod=CONTINUOUS
  state Operation
    state CarVisibility [parallel]
      settings: executionOrder=1
      state NoCar
        entry: car=0;
      state Car
        entry: car=1;
      (default) -> NoCar
      NoCar -> Car : [traffic_state==1]
      Car -> NoCar : [traffic_state==0]
    state DriverOperation [parallel]
      settings: executionOrder=2
      state Main
      (default) -> Main : {i=1;}
      Main -> (junction 22) : schedule[image_request]
      (junction 22) -> Main [order 2] : {image.data=0;
          | send(image);i = i + 1;}
      (junction 22) -> Main [order 1] : [(car==1)&&(blurryness(i)==1)]
          | {image.data=1;i = i + 1;send(image);}
  data: image_request input; traffic_state input; blurryness input; image output; car local; i local; schedule input

== stateflow chart iot_casestudy_1_32/CameraDriver25 ==
  settings: updateMethod=CONTINUOUS
  state Operation
    state CarVisibility [parallel]
      settings: executionOrder=1
      state NoCar
        entry: car=0;
      state Car
        entry: car=1;
      (default) -> NoCar
      NoCar -> Car : [traffic_state==1]
      Car -> NoCar : [traffic_state==0]
    state DriverOperation [parallel]
      settings: executionOrder=2
      state Main
      (default) -> Main : {i=1;}
      Main -> (junction 22) : schedule
          | [image_request]
      (junction 22) -> Main [order 1] : [(car==1)&&(blurryness(i)==1)]
          | {image.data=1;send(image);i = i + 1;}
      (junction 22) -> Main [order 2] : {image.data=0;
          | send(image);i = i + 1;}
  data: image_request input; traffic_state input; blurryness input; image output; car local; i local; schedule input

== stateflow chart iot_casestudy_1_32/CameraDriver26 ==
  settings: updateMethod=CONTINUOUS
  state Operation
    state CarVisibility [parallel]
      settings: executionOrder=1
      state NoCar
        entry: car=0;
      state Car
        entry: car=1;
      (default) -> NoCar
      NoCar -> Car : [traffic_state==1]
      Car -> NoCar : [traffic_state==0]
    state DriverOperation [parallel]
      settings: executionOrder=2
      state Main
      (default) -> Main : {i=1;}
      Main -> (junction 22) : schedule[image_request]
      (junction 22) -> Main [order 2] : {image.data=0;
          | send(image);i = i + 1;}
      (junction 22) -> Main [order 1] : [(car==1)&&(blurryness(i)==1)]
          | {image.data=1;i = i + 1;send(image);}
  data: image_request input; traffic_state input; blurryness input; image output; car local; i local; schedule input

== stateflow chart iot_casestudy_1_32/CameraDriver27 ==
  settings: updateMethod=CONTINUOUS
  state Operation
    state CarVisibility [parallel]
      settings: executionOrder=1
      state NoCar
        entry: car=0;
      state Car
        entry: car=1;
      (default) -> NoCar
      NoCar -> Car : [traffic_state==1]
      Car -> NoCar : [traffic_state==0]
    state DriverOperation [parallel]
      settings: executionOrder=2
      state Main
      (default) -> Main : {i=1;}
      Main -> (junction 22) : schedule
          | [image_request]
      (junction 22) -> Main [order 1] : [(car==1)&&(blurryness(i)==1)]
          | {image.data=1;send(image);i = i + 1;}
      (junction 22) -> Main [order 2] : {image.data=0;
          | send(image);i = i + 1;}
  data: image_request input; traffic_state input; blurryness input; image output; car local; i local; schedule input

== stateflow chart iot_casestudy_1_32/CameraDriver28 ==
  settings: updateMethod=CONTINUOUS
  state Operation
    state CarVisibility [parallel]
      settings: executionOrder=1
      state NoCar
        entry: car=0;
      state Car
        entry: car=1;
      (default) -> NoCar
      NoCar -> Car : [traffic_state==1]
      Car -> NoCar : [traffic_state==0]
    state DriverOperation [parallel]
      settings: executionOrder=2
      state Main
      (default) -> Main : {i=1;}
      Main -> (junction 22) : schedule[image_request]
      (junction 22) -> Main [order 2] : {image.data=0;
          | send(image);i = i + 1;}
      (junction 22) -> Main [order 1] : [(car==1)&&(blurryness(i)==1)]
          | {image.data=1;i = i + 1;send(image);}
  data: image_request input; traffic_state input; blurryness input; image output; car local; i local; schedule input

== stateflow chart iot_casestudy_1_32/CameraDriver29 ==
  settings: updateMethod=CONTINUOUS
  state Operation
    state CarVisibility [parallel]
      settings: executionOrder=1
      state NoCar
        entry: car=0;
      state Car
        entry: car=1;
      (default) -> NoCar
      NoCar -> Car : [traffic_state==1]
      Car -> NoCar : [traffic_state==0]
    state DriverOperation [parallel]
      settings: executionOrder=2
      state Main
      (default) -> Main : {i=1;}
      Main -> (junction 22) : schedule
          | [image_request]
      (junction 22) -> Main [order 1] : [(car==1)&&(blurryness(i)==1)]
          | {image.data=1;send(image);i = i + 1;}
      (junction 22) -> Main [order 2] : {image.data=0;
          | send(image);i = i + 1;}
  data: image_request input; traffic_state input; blurryness input; image output; car local; i local; schedule input

== stateflow chart iot_casestudy_1_32/CameraDriver30 ==
  settings: updateMethod=CONTINUOUS
  state Operation
    state CarVisibility [parallel]
      settings: executionOrder=1
      state NoCar
        entry: car=0;
      state Car
        entry: car=1;
      (default) -> NoCar
      NoCar -> Car : [traffic_state==1]
      Car -> NoCar : [traffic_state==0]
    state DriverOperation [parallel]
      settings: executionOrder=2
      state Main
      (default) -> Main : {i=1;}
      Main -> (junction 22) : schedule[image_request]
      (junction 22) -> Main [order 2] : {image.data=0;
          | send(image);i = i + 1;}
      (junction 22) -> Main [order 1] : [(car==1)&&(blurryness(i)==1)]
          | {image.data=1;i = i + 1;send(image);}
  data: image_request input; traffic_state input; blurryness input; image output; car local; i local; schedule input

== stateflow chart iot_casestudy_1_32/CameraDriver31 ==
  settings: updateMethod=CONTINUOUS
  state Operation
    state CarVisibility [parallel]
      settings: executionOrder=1
      state NoCar
        entry: car=0;
      state Car
        entry: car=1;
      (default) -> NoCar
      NoCar -> Car : [traffic_state==1]
      Car -> NoCar : [traffic_state==0]
    state DriverOperation [parallel]
      settings: executionOrder=2
      state Main
      (default) -> Main : {i=1;}
      Main -> (junction 22) : schedule
          | [image_request]
      (junction 22) -> Main [order 1] : [(car==1)&&(blurryness(i)==1)]
          | {image.data=1;send(image);i = i + 1;}
      (junction 22) -> Main [order 2] : {image.data=0;
          | send(image);i = i + 1;}
  data: image_request input; traffic_state input; blurryness input; image output; car local; i local; schedule input

== stateflow chart iot_casestudy_1_32/CameraScheduler16 ==
  settings: updateMethod=CONTINUOUS  executeAtInitialization=1
  state Main
    entry:
    dt=timer_array[i];
  (default) -> Main : {i=1;dt=0;}
  Main -> Main : after(dt,msec){i=i+1;send(schedule_driver);send(schedule_control);}
  data: timer_array input; schedule_driver output double; schedule_control output double; dt local double; dt2 local double; i output double =0.0

== stateflow chart iot_casestudy_1_32/CameraScheduler17 ==
  settings: updateMethod=CONTINUOUS  executeAtInitialization=1
  state Main
    entry:
    dt=timer_array[i];
  (default) -> Main : {i=0;dt=0;}
  Main -> Main : after(dt,msec){i=i+1;send(schedule_driver);send(schedule_control);}
  data: timer_array input; i local double; schedule_driver output double; schedule_control output double; dt local double

== stateflow chart iot_casestudy_1_32/CameraScheduler18 ==
  settings: updateMethod=CONTINUOUS  executeAtInitialization=1
  state Main
    entry:
    dt=timer_array[i];
  (default) -> Main : {i=1;dt=0;}
  Main -> Main : after(dt,msec){i=i+1;send(schedule_driver);send(schedule_control);}
  data: timer_array input; schedule_driver output double; schedule_control output double; dt local double; dt2 local double; i local double =0.0

== stateflow chart iot_casestudy_1_32/CameraScheduler19 ==
  settings: updateMethod=CONTINUOUS  executeAtInitialization=1
  state Main
    entry:
    dt=timer_array[i];
  (default) -> Main : {i=0;dt=0;}
  Main -> Main : after(dt,msec){i=i+1;send(schedule_driver);send(schedule_control);}
  data: timer_array input; i local double; schedule_driver output double; schedule_control output double; dt local double

== stateflow chart iot_casestudy_1_32/CameraScheduler20 ==
  settings: updateMethod=CONTINUOUS  executeAtInitialization=1
  state Main
    entry:
    dt=timer_array[i];
  (default) -> Main : {i=1;dt=0;}
  Main -> Main : after(dt,msec){i=i+1;send(schedule_driver);send(schedule_control);}
  data: timer_array input; schedule_driver output double; schedule_control output double; dt local double; dt2 local double; i local double =0.0

== stateflow chart iot_casestudy_1_32/CameraScheduler21 ==
  settings: updateMethod=CONTINUOUS  executeAtInitialization=1
  state Main
    entry:
    dt=timer_array[i];
  (default) -> Main : {i=0;dt=0;}
  Main -> Main : after(dt,msec){i=i+1;send(schedule_driver);send(schedule_control);}
  data: timer_array input; i local double; schedule_driver output double; schedule_control output double; dt local double

== stateflow chart iot_casestudy_1_32/CameraScheduler22 ==
  settings: updateMethod=CONTINUOUS  executeAtInitialization=1
  state Main
    entry:
    dt=timer_array[i];
  (default) -> Main : {i=1;dt=0;}
  Main -> Main : after(dt,msec){i=i+1;send(schedule_driver);send(schedule_control);}
  data: timer_array input; schedule_driver output double; schedule_control output double; dt local double; dt2 local double; i local double =0.0

== stateflow chart iot_casestudy_1_32/CameraScheduler23 ==
  settings: updateMethod=CONTINUOUS  executeAtInitialization=1
  state Main
    entry:
    dt=timer_array[i];
  (default) -> Main : {i=0;dt=0;}
  Main -> Main : after(dt,msec){i=i+1;send(schedule_driver);send(schedule_control);}
  data: timer_array input; i local double; schedule_driver output double; schedule_control output double; dt local double

== stateflow chart iot_casestudy_1_32/CameraScheduler24 ==
  settings: updateMethod=CONTINUOUS  executeAtInitialization=1
  state Main
    entry:
    dt=timer_array[i];
  (default) -> Main : {i=1;dt=0;}
  Main -> Main : after(dt,msec){i=i+1;send(schedule_driver);send(schedule_control);}
  data: timer_array input; schedule_driver output double; schedule_control output double; dt local double; dt2 local double; i output double =0.0

== stateflow chart iot_casestudy_1_32/CameraScheduler25 ==
  settings: updateMethod=CONTINUOUS  executeAtInitialization=1
  state Main
    entry:
    dt=timer_array[i];
  (default) -> Main : {i=0;dt=0;}
  Main -> Main : after(dt,msec){i=i+1;send(schedule_driver);send(schedule_control);}
  data: timer_array input; i local double; schedule_driver output double; schedule_control output double; dt local double

== stateflow chart iot_casestudy_1_32/CameraScheduler26 ==
  settings: updateMethod=CONTINUOUS  executeAtInitialization=1
  state Main
    entry:
    dt=timer_array[i];
  (default) -> Main : {i=1;dt=0;}
  Main -> Main : after(dt,msec){i=i+1;send(schedule_driver);send(schedule_control);}
  data: timer_array input; schedule_driver output double; schedule_control output double; dt local double; dt2 local double; i output double =0.0

== stateflow chart iot_casestudy_1_32/CameraScheduler27 ==
  settings: updateMethod=CONTINUOUS  executeAtInitialization=1
  state Main
    entry:
    dt=timer_array[i];
  (default) -> Main : {i=0;dt=0;}
  Main -> Main : after(dt,msec){i=i+1;send(schedule_driver);send(schedule_control);}
  data: timer_array input; i local double; schedule_driver output double; schedule_control output double; dt local double

== stateflow chart iot_casestudy_1_32/CameraScheduler28 ==
  settings: updateMethod=CONTINUOUS  executeAtInitialization=1
  state Main
    entry:
    dt=timer_array[i];
  (default) -> Main : {i=1;dt=0;}
  Main -> Main : after(dt,msec){i=i+1;send(schedule_driver);send(schedule_control);}
  data: timer_array input; schedule_driver output double; schedule_control output double; dt local double; dt2 local double; i output double =0.0
